simulink model "sampleModel1952"  (R2023a)
settings: Solver=VariableStepAuto  StartTime=0.0  StopTime=10.0  RelTol=1e-3
libraries: hdlsllib x7, simulink x5
settings Model: Creator=user1  LastModifiedBy=user1

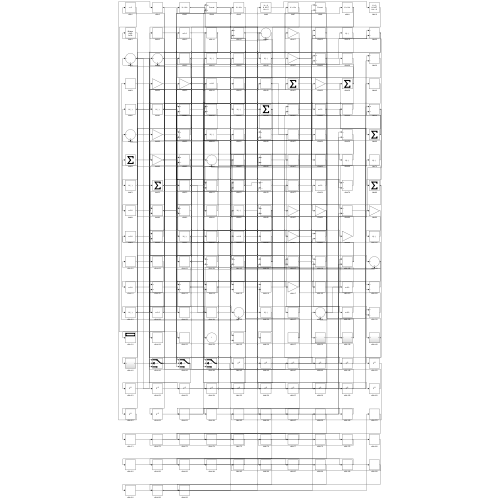
[thumbnail: Simulink's stored preview of the top-level diagram]
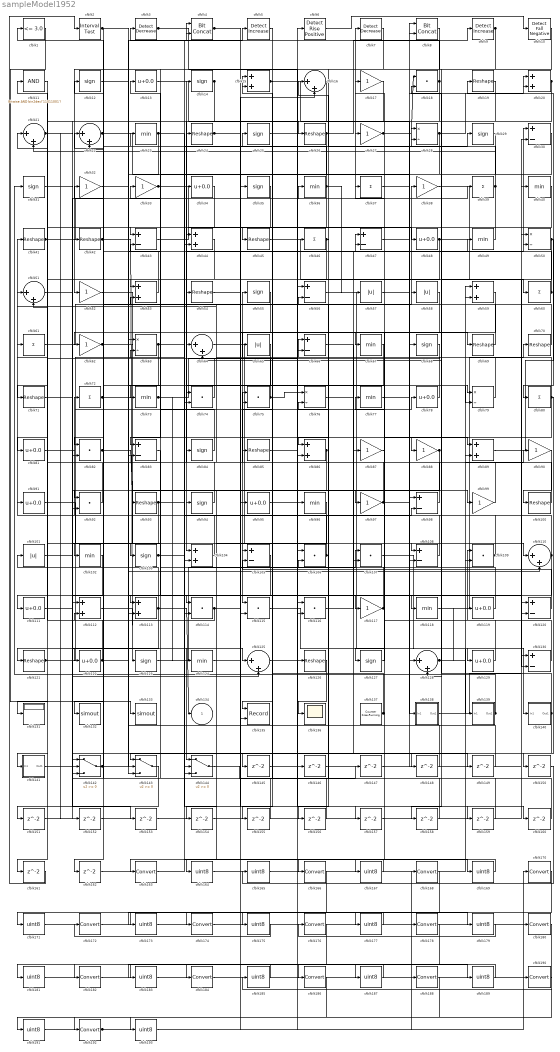
== system sampleModel1952 ==
  cfblk1 : hdlsllib/Logic and Bit Operations/Compare To Constant  relop=<=  const=3.0  OutDataTypeStr=boolean
  cfblk10 : hdlsllib/Logic and Bit Operations/Detect Fall Negative  vinit=0  OutDataTypeStr=boolean
  cfblk{19,24,26,41..42,45,54,69..71,85,93,100,121,126} (15 alike) : Reshape
  cfblk{57..58,65,101} (4 alike) : Abs  SaturateOnIntegerOverflow=off
  cfblk{23,36,40,49,67,73,77,96,102,118,124} (11 alike) : MinMax
  cfblk{12,14,25,29,31,35,55,68,84,94,103,123,127} (13 alike) : Signum
  cfblk{15,20,44,53,59,86,89,104,112..113} (10 alike) : Sum
  cfblk{30,43,47,56,66,83,98,105,108,120,130} (11 alike) : Sum  Inputs=+-
  cfblk{18,74..75,82,92,106..107,109,114..116} (11 alike) : DotProduct  OutDataTypeStr=Inherit: Inherit via internal rule
  cfblk11 : simulink/Logic and Bit Operations/Bitwise Operator  logicop=AND  UseBitMask=on  BitMask=bin2dec('11011001')  BitMaskRealWorld=Stored Integer
      settings: LibrarySourceBlock=|
      | hdlsllib/Logic and Bit
      | Operations/Bitwise
      | Operator
  cfblk{16,21..22,51,64,110,125,128} (8 alike) : Sum  Inputs=|++
  cfblk{13,34,48,78,81,91,95,111,119,122,129} (11 alike) : Bias  Bias=0.0  SaturateOnIntegerOverflow=off
  cfblk{17,27,32..33,38,52,62,87..88,90,97,99,117} (13 alike) : Gain
  cfblk131 : Display
  cfblk132 : ToWorkspace  VariableName=simout  SaveFormat=Timeseries  SampleTime=-1
  cfblk133 : ToWorkspace  VariableName=simout  SaveFormat=Timeseries  SampleTime=-1
  cfblk135 : Record  FileSettingsInternal="{\"entries\":[{\"content\":{\"excelSettings\":{\"content\":{},\"type\":\"Streamout.ExcelSettings\"}},\"type\":\"Streamout.FileSettingStorage\",\"uuid\":\"\"}],\"packageUris\":[\"http:\\/\\/schema.mathworks.com\\/mf0\\/streamout_blocks\\/R2020a\"],\"version\":\"1.0\"}"  Layout=[1 1]  SignalsInternal="{\"entries\":[{\"content\":{\"signals\":[{\"content\":{\"blockPath\":[],\"dimensions\":[1],\"domain\":\"\",\"lineColor\":\"#a2142f\",\"plots\":[1],\"port\":1,\"signalID\":5446,\"signalName\":\"XY Graph:1\"},\"type\":\"RecordBlkView.Signal\",\"uuid\":\"\"},{\"content\":{\"blockPath\":[],\"dimensions\":[1],\"domain\":\"\",\"lineColor\":\"#139fff\",\"plots\":[1],\"port\":2,\"signalID\":5449,\"signalName\":\"XY Graph:2\"},\"type\":\"RecordBlkView.Signal\",\"uuid\":\"\"}]},\"type\":\"RecordBlkView.InputSignals\",\"uuid\":\"\"}],\"packageUris\":[\"http:\\/\\/schema.mathworks.com\\/mf0\\/streamout_blocks\\/R2020a\"],\"version\":\"1.0\"}"  VisualizationBindings="{\"xyplotplugin\":{\"info\":[{\"series\":[{\"bindingParametersList\":[{\"parameter\":\"X-Axis\",\"signalID\":5446,\"signalName\":\"XY Graph:1\"},{\"parameter\":\"Y-Axis\",\"signalID\":5449,\"signalName\":\"XY Graph:2\"}],\"seriesID\":23493}],\"subplotID\":1}]}}"  CompatibilityTag=XY  st=-1
  cfblk136 : Scope
  cfblk137 : hdlsllib/Sources/Counter Free-Running  NumBits=16  tsamp=-1
  cfblk138 : Subsystem
      settings: LibrarySourceBlock=|
      | hdlsllib/Ports &
      | Subsystems/Subsystem
  cfblk139 : Subsystem
      settings: LibrarySourceBlock=|
      | hdlsllib/Ports &
      | Subsystems/Subsystem
  cfblk140 : Subsystem
      settings: LibrarySourceBlock=|
      | hdlsllib/Ports &
      | Subsystems/Subsystem
  cfblk141 : Subsystem
      settings: LibrarySourceBlock=|
      | hdlsllib/Ports &
      | Subsystems/Subsystem
  cfblk142 : Switch  SaturateOnIntegerOverflow=off  InputSameDT=off
  cfblk143 : Switch  SaturateOnIntegerOverflow=off  InputSameDT=off
  cfblk144 : Switch  SaturateOnIntegerOverflow=off  InputSameDT=off
  cfblk{145..162} (18 alike) : Delay  SampleTime=1
  cfblk{163,166,168,170,172,174,176,178,180,182,184,186,188,190,192} (15 alike) : DataTypeConversion  SaturateOnIntegerOverflow=off  RndMeth=Floor
  cfblk{164..165,167,169,171,173,175,177,179,181,183,185,187,189,191,193} (16 alike) : DataTypeConversion  OutDataTypeStr=uint8  SaturateOnIntegerOverflow=off  RndMeth=Floor
  cfblk2 : hdlsllib/Logic and Bit Operations/Interval Test  IntervalClosedRight=on  uplimit=0.5  IntervalClosedLeft=on  lowlimit=-0.5  OutDataTypeStr=boolean
  cfblk{28,50,63,76,79} (5 alike) : Product  Inputs=*/  RndMeth=Zero  SaturateOnIntegerOverflow=on
  cfblk3 : simulink/Logic and Bit Operations/Detect Decrease  vinit=0.0  OutDataTypeStr=boolean
      settings: LibrarySourceBlock=|
      | hdlsllib/Logic and Bit
      | Operations/Detect
      | Decrease
  cfblk{37,39,46,60..61,72,80} (7 alike) : Sum  Inputs=+
  cfblk4 : hdlsllib/Logic and Bit Operations/Bit Concat  numInputs=2
  cfblk5 : simulink/Logic and Bit Operations/Detect Increase  vinit=0.0  OutDataTypeStr=boolean
      settings: LibrarySourceBlock=|
      | hdlsllib/Logic and Bit
      | Operations/Detect
      | Increase
  cfblk6 : hdlsllib/Logic and Bit Operations/Detect Rise Positive  vinit=0  OutDataTypeStr=boolean
  cfblk7 : simulink/Logic and Bit Operations/Detect Decrease  vinit=0.0  OutDataTypeStr=boolean
      settings: LibrarySourceBlock=|
      | hdlsllib/Logic and Bit
      | Operations/Detect
      | Decrease
  cfblk8 : hdlsllib/Logic and Bit Operations/Bit Concat  numInputs=2
  cfblk9 : simulink/Logic and Bit Operations/Detect Increase  vinit=0.0  OutDataTypeStr=boolean
      settings: LibrarySourceBlock=|
      | hdlsllib/Logic and Bit
      | Operations/Detect
      | Increase
  cfblk134 : Outport  VectorParamsAs1DForOutWhenUnconnected=off
  wires:
  cfblk13/1 -> cfblk26/1
  cfblk56/1 -> cfblk129/1
  cfblk62/1 -> cfblk97/1, cfblk47/2
  cfblk118/1 -> cfblk70/1
  cfblk60/1 -> cfblk30/1, cfblk15/1
  cfblk106/1 -> cfblk41/1, cfblk76/2
  cfblk55/1 -> cfblk115/1
  cfblk10/1 -> cfblk52/1
  cfblk84/1 -> cfblk33/1
  cfblk124/1 -> cfblk35/1
  cfblk61/1 -> cfblk38/1
  cfblk28/1 -> cfblk104/1, cfblk20/1
  cfblk139/1(Out1) -> cfblk31/1, cfblk64/2
  cfblk52/1 -> cfblk104/2
  cfblk42/1 -> cfblk123/1, cfblk79/2, cfblk34/1
  cfblk22/1 -> cfblk68/1, cfblk132/1
  cfblk70/1 -> cfblk32/1
  cfblk86/1 -> cfblk103/1, cfblk164/1
  cfblk1/1 -> cfblk133/1
  cfblk94/1 -> cfblk14/1
  cfblk7/1 -> cfblk86/1
  cfblk88/1 -> cfblk94/1, cfblk108/2, cfblk142/3
  cfblk17/1 -> cfblk64/1
  cfblk89/1 -> cfblk19/1
  cfblk140/1(Out1) -> cfblk143/1, cfblk18/2
  cfblk43/1 -> cfblk48/1
  cfblk82/1 -> cfblk93/1, cfblk4/2
  cfblk97/1 -> cfblk22/1, cfblk29/1
  cfblk18/1 -> cfblk3/1, cfblk82/2
  cfblk112/1 -> cfblk144/1
  cfblk2/1 -> cfblk62/1, cfblk116/2
  cfblk72/1 -> cfblk89/1, cfblk4/1
  cfblk122/1 -> cfblk11/1, cfblk78/1
  cfblk108/1 -> cfblk66/1
  cfblk45/1 -> cfblk60/1
  cfblk120/1 -> cfblk25/1
  cfblk138/1(Out1) -> cfblk40/1
  cfblk14/1 -> cfblk71/1, cfblk92/2
  cfblk19/1 -> cfblk88/1
  cfblk5/1 -> cfblk45/1
  cfblk64/1 -> cfblk108/1
  cfblk33/1 -> cfblk106/1, cfblk145/1
  cfblk121/1 -> cfblk58/1, cfblk36/1
  cfblk74/1 -> cfblk21/1
  cfblk41/1 -> cfblk7/1, cfblk125/2
  cfblk29/1 -> cfblk73/1
  cfblk107/1 -> cfblk140/1(In1)
  cfblk69/1 -> cfblk24/1
  cfblk127/1 -> cfblk77/1
  cfblk79/1 -> cfblk51/1
  cfblk123/1 -> cfblk107/1
  cfblk20/1 -> cfblk53/1, cfblk82/1
  cfblk104/1 -> cfblk72/1
  cfblk81/1 -> cfblk56/1
  cfblk40/1 -> cfblk122/1
  cfblk57/1 -> cfblk8/1
  cfblk78/1 -> cfblk55/1
  cfblk3/1 -> cfblk126/1, cfblk46/1
  cfblk36/1 -> cfblk1/1, cfblk114/2, cfblk57/1
  cfblk26/1 -> cfblk135/1, cfblk9/1
  cfblk83/1 -> cfblk113/1
  cfblk128/1 -> cfblk90/1, cfblk119/1
  cfblk80/1 -> cfblk127/1, cfblk28/2, cfblk150/1
  cfblk137/1 -> cfblk44/1, cfblk91/1
  cfblk73/1 -> cfblk6/1, cfblk124/1
  cfblk98/1 -> cfblk17/1
  cfblk16/1 -> cfblk66/2
  cfblk115/1 -> cfblk139/1(In1)
  cfblk129/1 -> cfblk37/1
  cfblk63/1 -> cfblk5/1, cfblk92/1
  cfblk50/1 -> cfblk80/1, cfblk158/1
  cfblk130/1 -> cfblk109/1
  cfblk39/1 -> cfblk143/2, cfblk21/2, cfblk16/1
  cfblk91/1 -> cfblk105/1
  cfblk75/1 -> cfblk65/1, cfblk76/1
  cfblk53/1 -> cfblk12/1
  cfblk141/1(Out1) -> cfblk112/1
  cfblk67/1 -> cfblk115/2
  cfblk9/1 -> cfblk128/2, cfblk83/1
  cfblk93/1 -> cfblk118/1, cfblk131/1
  cfblk99/1 -> cfblk54/1
  cfblk38/1 -> cfblk120/1
  cfblk21/1 -> cfblk144/3, cfblk110/1, cfblk152/1
  cfblk49/1 -> cfblk42/1
  cfblk105/1 -> cfblk143/3
  cfblk111/1 -> cfblk39/1
  cfblk126/1 -> cfblk136/1
  cfblk92/1 -> cfblk61/1
  cfblk24/1 -> cfblk117/1, cfblk107/2
  cfblk47/1 -> cfblk120/2
  cfblk11/1 -> cfblk81/1
  cfblk31/1 -> cfblk125/1
  cfblk35/1 -> cfblk102/1
  cfblk76/1 -> cfblk87/1
  cfblk8/1 -> cfblk113/2
  cfblk71/1 -> cfblk114/1
  cfblk4/1 -> cfblk67/1, cfblk157/1
  cfblk100/1 -> cfblk75/1
  cfblk114/1 -> cfblk112/2, cfblk16/2
  cfblk34/1 -> cfblk51/2
  cfblk87/1 -> cfblk27/1
  cfblk37/1 -> cfblk79/1
  cfblk77/1 -> cfblk8/2
  cfblk68/1 -> cfblk63/2
  cfblk116/1 -> cfblk50/2
  cfblk117/1 -> cfblk56/2, cfblk53/2
  cfblk54/1 -> cfblk69/1
  cfblk30/1 -> cfblk43/1
  cfblk109/1 -> cfblk13/1, cfblk23/1
  cfblk23/1 -> cfblk99/1, cfblk83/2
  cfblk65/1 -> cfblk84/1
  cfblk113/1 -> cfblk134/1, cfblk141/1(In1), cfblk98/2, cfblk101/1
  cfblk32/1 -> cfblk74/1
  cfblk125/1 -> cfblk96/1
  cfblk90/1 -> cfblk100/1
  cfblk27/1 -> cfblk18/1, cfblk20/2
  cfblk15/1 -> cfblk138/1(In1), cfblk155/1
  cfblk46/1 -> cfblk111/1, cfblk156/1
  cfblk95/1 -> cfblk47/1
  cfblk48/1 -> cfblk130/2, cfblk144/2
  cfblk6/1 -> cfblk10/1
  cfblk119/1 -> cfblk85/1
  cfblk103/1 -> cfblk28/1, cfblk159/1
  cfblk12/1 -> cfblk74/2
  cfblk142/1 -> cfblk49/1, cfblk110/2
  cfblk44/1 -> cfblk121/1
  cfblk110/1 -> cfblk135/2, cfblk105/2, cfblk15/2
  cfblk145/1 -> cfblk30/2
  cfblk25/1 -> cfblk146/1
  cfblk146/1 -> cfblk109/2
  cfblk144/1 -> cfblk147/1
  cfblk147/1 -> cfblk128/1
  cfblk66/1 -> cfblk148/1
  cfblk148/1 -> cfblk98/1
  cfblk101/1 -> cfblk149/1
  cfblk149/1 -> cfblk63/1
  cfblk143/1 -> cfblk151/1
  cfblk151/1 -> cfblk142/1
  cfblk152/1 -> cfblk86/2
  cfblk51/1 -> cfblk153/1
  cfblk153/1 -> cfblk50/1
  cfblk96/1 -> cfblk154/1
  cfblk154/1 -> cfblk130/1
  cfblk155/1 -> cfblk43/2
  cfblk156/1 -> cfblk142/2
  cfblk157/1 -> cfblk89/2
  cfblk158/1 -> cfblk106/2
  cfblk159/1 -> cfblk75/2
  cfblk85/1 -> cfblk160/1
  cfblk160/1 -> cfblk22/2
  cfblk102/1 -> cfblk161/1
  cfblk161/1 -> cfblk2/1
  cfblk58/1 -> cfblk162/1
  cfblk162/1 -> cfblk44/2
  cfblk164/1 -> cfblk59/1
  cfblk150/1 -> cfblk165/1
  cfblk165/1 -> cfblk59/2
  cfblk59/1 -> cfblk167/1
  cfblk167/1 -> cfblk163/1
  cfblk163/1 -> cfblk169/1
  cfblk169/1 -> cfblk166/1
  cfblk166/1 -> cfblk171/1
  cfblk171/1 -> cfblk168/1
  cfblk168/1 -> cfblk173/1
  cfblk173/1 -> cfblk170/1
  cfblk170/1 -> cfblk175/1
  cfblk175/1 -> cfblk172/1
  cfblk172/1 -> cfblk177/1
  cfblk177/1 -> cfblk174/1
  cfblk174/1 -> cfblk179/1
  cfblk179/1 -> cfblk176/1
  cfblk176/1 -> cfblk181/1
  cfblk181/1 -> cfblk178/1
  cfblk178/1 -> cfblk183/1
  cfblk183/1 -> cfblk180/1
  cfblk180/1 -> cfblk185/1
  cfblk185/1 -> cfblk182/1
  cfblk182/1 -> cfblk187/1
  cfblk187/1 -> cfblk184/1
  cfblk184/1 -> cfblk189/1
  cfblk189/1 -> cfblk186/1
  cfblk190/1 -> cfblk192/1
  cfblk186/1 -> cfblk191/1
  cfblk191/1 -> cfblk188/1
  cfblk192/1 -> cfblk116/1, cfblk95/1
  cfblk188/1 -> cfblk193/1
  cfblk193/1 -> cfblk190/1

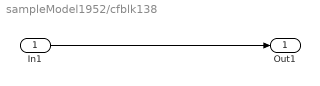
== system sampleModel1952/cfblk138 ==
  In1 : Inport
  Out1 : Outport
  wires:
  In1/1 -> Out1/1

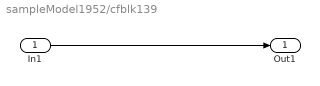
== system sampleModel1952/cfblk139 ==
  In1 : Inport
  Out1 : Outport
  wires:
  In1/1 -> Out1/1

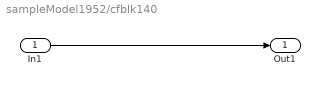
== system sampleModel1952/cfblk140 ==
  In1 : Inport
  Out1 : Outport
  wires:
  In1/1 -> Out1/1

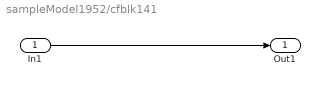
== system sampleModel1952/cfblk141 ==
  In1 : Inport
  Out1 : Outport
  wires:
  In1/1 -> Out1/1
